simulink model "Regelungsansatz_aus_RLM"  (R2016b)
settings: Solver=VariableStepAuto  StartTime=0.0  StopTime=10.0  RelTol=1e-3
settings Model: Creator=nicol  LastModifiedBy=nicol

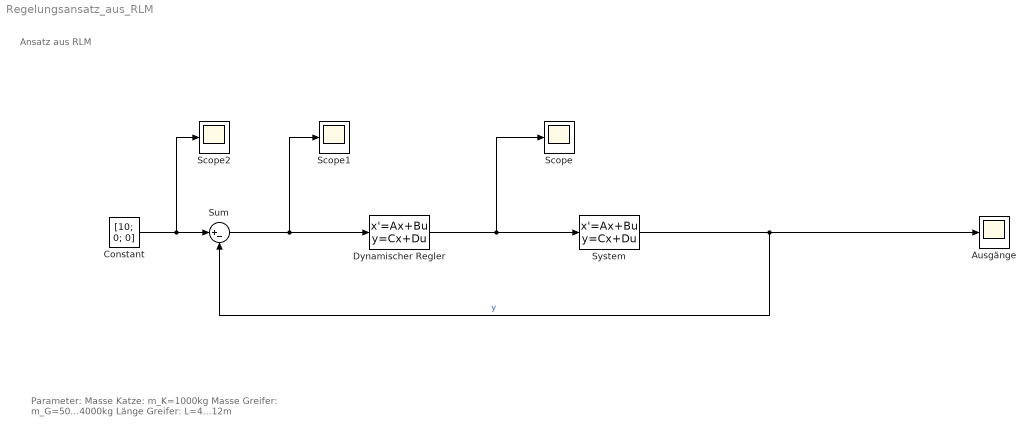
== system Regelungsansatz_aus_RLM ==
  note: Ansatz aus RLM
  note: Parameter:
      | Masse Katze: m_K=1000kg
      | Masse Greifer: m_G=50...4000kg
      | Länge Greifer: L=4...12m
  Ausgänge : Scope
  Constant : Constant  Value=[10; 0; 0]  VectorParams1D=off
  Dynamischer Regler : StateSpace  A=-0.6  B=[7.2 25.4 -306.2]  C=1000.7  D=[144.7 10294.8 -10032.5]  X0=0
  Scope : Scope
  Scope1 : Scope
  Scope2 : Scope
  Sum : Sum  Inputs=|+-
  System : StateSpace  A=[0 1 0 0; 0 0 39.24 0; 0 0 0 1; 0 0 -4.0875 0]  B=[0; 0.001; 0; -0.000083333]  C=[1 0 0 0; 0 1 0 0; 0 0 1 0]  D=[0; 0; 0]  X0=0
  wires:
  System/1 -> Sum/2, Ausgänge/1  "y"
  Constant/1 -> Scope2/1, Sum/1
  Dynamischer Regler/1 -> Scope/1, System/1
  Sum/1 -> Scope1/1, Dynamischer Regler/1
